simulink model "motor_unit"  (Simulink 7.7)
settings: Solver=ode1  StartTime=0.0  StopTime=1  FixedStep=.001  RelTol=1e-3
settings Model: Creator=minos_niu  LastModifiedBy=minos_niu

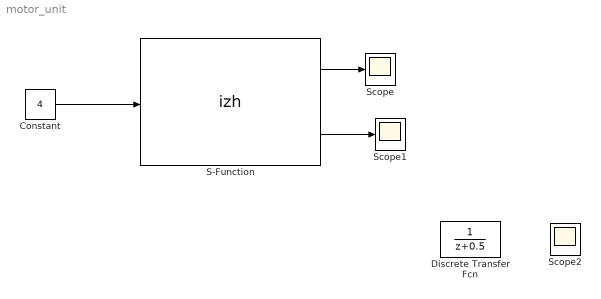
== system motor_unit ==
  Constant : Constant  Value=4
  Discrete Transfer Fcn : DiscreteTransferFcn  SampleTime=-1
  S-Function : S-Function  FunctionName=izh  Parameters=[0.02 0.2 -65.0 6.0] [-70.0 -14.0]  EnableBusSupport=off
      mask Display:
      | port_label('input', 1, 'syn curr');
      | port_label('output', 1, 'action potential');
      | port_label('output', 2, 'spike');
      | disp('Izhi Neuron \n(S-Function)')
  Scope : Scope
  Scope1 : Scope
  Scope2 : Scope
      settings: SaveName=ScopeData2
  wires:
  Constant/1 -> S-Function/1
  S-Function/1 -> Scope/1
  S-Function/2 -> Scope1/1
